simulink model "GNP"  (R2012b)
settings: Solver=ode3  StartTime=0.0  StopTime=sim_time  FixedStep=Ts  RelTol=1e-3
values from neighbouring files (symbols this model uses):
  education = 20    [simulate_gnp.m]
  population = 100000    [simulate_gnp.m]
  public_average_salary = 25000    [simulate_gnp.m]
  public_employees = 20000    [simulate_gnp.m]
  tax = 0.3    [simulate_gnp.m]
  unemployees = (population - public_employees - car_employees -     oil_employees - food_employees)/population    (= 0.45)    [simulate_gnp.m]
libraries: NeoFinansLibrary x3
settings Model: Creator=ägarenn  LastModifiedBy=ägarenn
settings DebuggingCC: SolverPrmCheckMsg=none

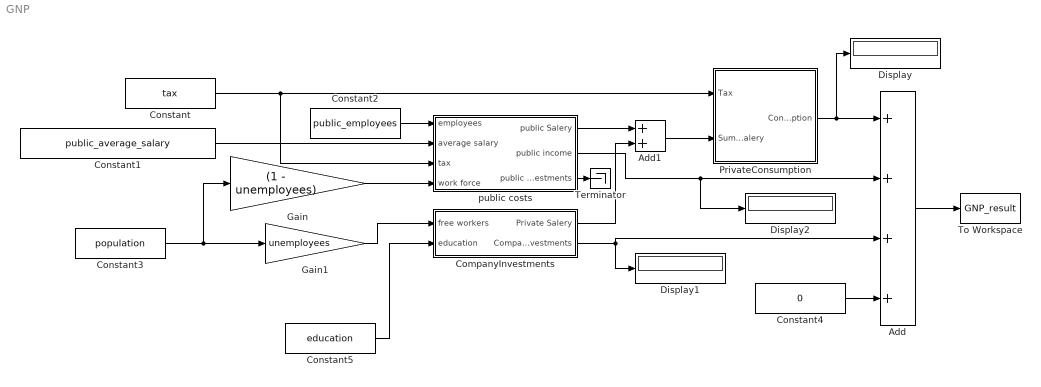
== system GNP ==
  Add : Sum  Inputs=++++
  Add1 : Sum
  CompanyInvestments : Subsystem
  Constant : Constant  Value=tax
  Constant1 : Constant  Value=public_average_salary
  Constant2 : Constant  Value=public_employees
  Constant3 : Constant  Value=population
  Constant4 : Constant  Value=0
  Constant5 : Constant  Value=education
  Display : Display
  Display1 : Display
  Display2 : Display
  Gain : Gain  Gain=(1 - unemployees)
  Gain1 : Gain  Gain=unemployees
  PrivateConsumption : Subsystem
  Terminator : Terminator
  To Workspace : ToWorkspace  VariableName=GNP_result  SampleTime=-1  SaveFormat=Timeseries
  public costs : Subsystem
  wires:
  Add/1 -> To Workspace/1
  CompanyInvestments/2(Company Investments) -> Add/3, Display1/1
  Add1/1 -> PrivateConsumption/2(SumSalery)
  public costs/1(public Salery) -> Add1/1
  CompanyInvestments/1(Private Salery) -> Add1/2
  public costs/2(public income) -> Display2/1, Add/2
  Constant/1 -> public costs/3(tax), PrivateConsumption/1(Tax)
  Constant1/1 -> public costs/2(average salary)
  Constant2/1 -> public costs/1(employees)
  Gain/1 -> public costs/4(work force)
  Constant3/1 -> Gain1/1, Gain/1
  Constant4/1 -> Add/4
  public costs/3(public investments) -> Terminator/1
  PrivateConsumption/1(Consumption) -> Display/1, Add/1
  Constant5/1 -> CompanyInvestments/2(education)
  Gain1/1 -> CompanyInvestments/1(free workers)

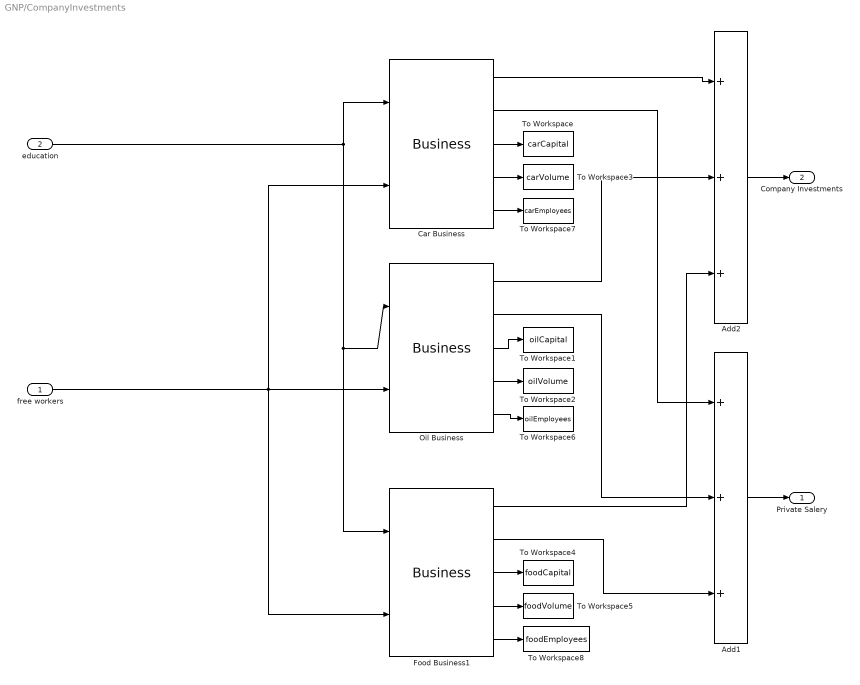
== system GNP/CompanyInvestments ==
  free workers : Inport
  education : Inport  Port=2
  Add1 : Sum  Inputs=+++
  Add2 : Sum  Inputs=+++
  Car Business : NeoFinansLibrary/Business  price=car_price  salary=car_salary  employees=car_employees  effectPerUnit=car_effect_unit  materialCost=car_material  productionCost=car_production  startCapital=10^10  KpEmployeeController=car_KpEmployeeController  KiEmployeeController=car_KiEmployeeController
  Food Business1 : NeoFinansLibrary/Business  price=food_price  salary=food_salary  employees=food_employees  effectPerUnit=food_effect_unit  materialCost=food_material  productionCost=food_production  startCapital=10^10  KpEmployeeController=food_KpEmployeeController  KiEmployeeController=food_KiEmployeeController
  Oil Business : NeoFinansLibrary/Business  price=oil_price  salary=oil_salary  employees=oil_employees  effectPerUnit=oil_effect_unit  materialCost=oil_material  productionCost=oil_production  startCapital=10^10  KpEmployeeController=oil_KpEmployeeController  KiEmployeeController=oil_KiEmployeeController
  To Workspace : ToWorkspace  VariableName=carCapital  SampleTime=-1  SaveFormat=Timeseries
  To Workspace1 : ToWorkspace  VariableName=oilCapital  SampleTime=-1  SaveFormat=Timeseries
  To Workspace2 : ToWorkspace  VariableName=oilVolume  SampleTime=-1  SaveFormat=Timeseries
  To Workspace3 : ToWorkspace  VariableName=carVolume  SampleTime=-1  SaveFormat=Timeseries
  To Workspace4 : ToWorkspace  VariableName=foodCapital  SampleTime=-1  SaveFormat=Timeseries
  To Workspace5 : ToWorkspace  VariableName=foodVolume  SampleTime=-1  SaveFormat=Timeseries
  To Workspace6 : ToWorkspace  VariableName=oilEmployees  SampleTime=-1  SaveFormat=Timeseries
  To Workspace7 : ToWorkspace  VariableName=carEmployees  SampleTime=-1  SaveFormat=Timeseries
  To Workspace8 : ToWorkspace  VariableName=foodEmployees  SampleTime=-1  SaveFormat=Timeseries
  Private Salery : Outport
  Company Investments : Outport  Port=2
  wires:
  Add2/1 -> Company Investments/1
  Car Business/1 -> Add2/1
  Add1/1 -> Private Salery/1
  Car Business/2 -> Add1/1
  education/1 -> Food Business1/1, Oil Business/1, Car Business/1
  Car Business/3 -> To Workspace/1
  Car Business/4 -> To Workspace3/1
  Oil Business/1 -> Add2/2
  Oil Business/2 -> Add1/2
  Oil Business/3 -> To Workspace1/1
  Oil Business/4 -> To Workspace2/1
  Food Business1/1 -> Add2/3
  Food Business1/2 -> Add1/3
  Food Business1/3 -> To Workspace4/1
  Food Business1/4 -> To Workspace5/1
  Oil Business/5 -> To Workspace6/1
  free workers/1 -> Food Business1/2, Car Business/2, Oil Business/2
  Car Business/5 -> To Workspace7/1
  Food Business1/5 -> To Workspace8/1

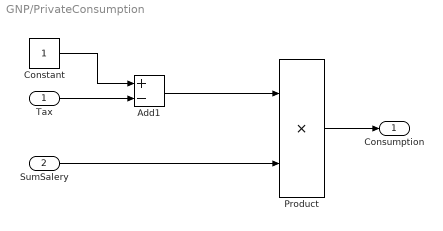
== system GNP/PrivateConsumption ==
  Tax : Inport
  SumSalery : Inport  Port=2
  Add1 : Sum  Inputs=+-
  Constant : Constant
  Product : Product  RndMeth=Zero
  Consumption : Outport
  wires:
  Product/1 -> Consumption/1
  Tax/1 -> Add1/2
  Add1/1 -> Product/1
  Constant/1 -> Add1/1
  SumSalery/1 -> Product/2

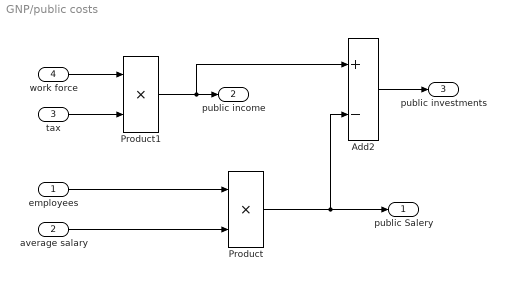
== system GNP/public costs ==
  employees : Inport
  average salary : Inport  Port=2
  tax : Inport  Port=3
  work force : Inport  Port=4
  Add2 : Sum  Inputs=+-
  Product : Product  RndMeth=Zero
  Product1 : Product  RndMeth=Zero
  public Salery : Outport
  public income : Outport  Port=2
  public investments : Outport  Port=3
  wires:
  Product/1 -> Add2/2, public Salery/1
  employees/1 -> Product/1
  average salary/1 -> Product/2
  work force/1 -> Product1/1
  tax/1 -> Product1/2
  Product1/1 -> Add2/1, public income/1
  Add2/1 -> public investments/1
